simulink model "TST_RailP_DD"  (R2016b)
settings: Solver=FixedStepDiscrete  StartTime=0.0  StopTime=simTime  FixedStep=sampleTime  RelTol=1e-3
values from neighbouring files (symbols this model uses):
  testCase = 1    [initTST_RailP_DD_001.m]    (also in initTST_RailP_DD_002.m = 2; initTST_RailP_DD_003.m = 3)
libraries: UnitTest_Lib x15, simulink x4
settings Model: Creator=liangyunbo  LastModifiedBy=liangyunbo
settings DebuggingCC: SignalRangeChecking=error

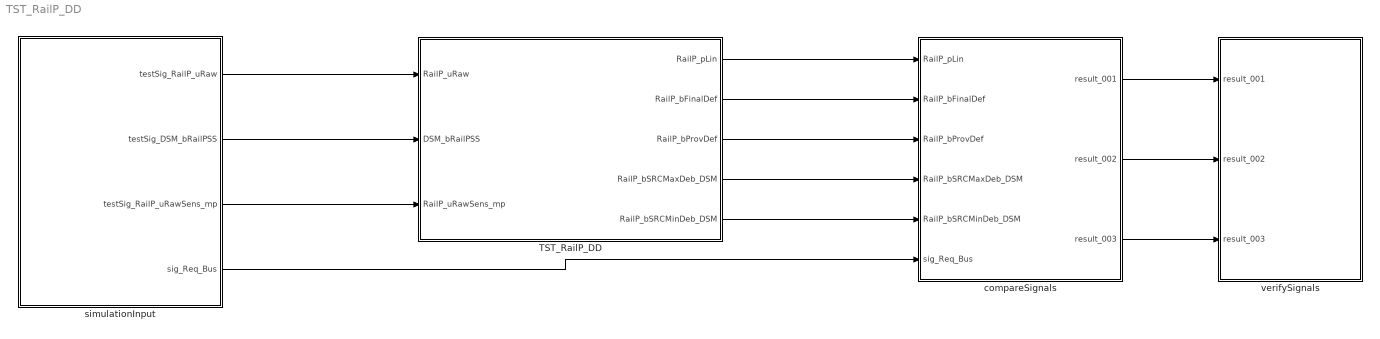
== system TST_RailP_DD ==
  TST_RailP_DD : Subsystem
  compareSignals : Subsystem
  simulationInput : Subsystem
  verifySignals : Subsystem
  wires:
  simulationInput/1(testSig_RailP_uRaw) -> TST_RailP_DD/1(RailP_uRaw)
  simulationInput/2(testSig_DSM_bRailPSS) -> TST_RailP_DD/2(DSM_bRailPSS)
  simulationInput/3(testSig_RailP_uRawSens_mp) -> TST_RailP_DD/3(RailP_uRawSens_mp)
  TST_RailP_DD/1(RailP_pLin) -> compareSignals/1(RailP_pLin)
  TST_RailP_DD/2(RailP_bFinalDef) -> compareSignals/2(RailP_bFinalDef)
  TST_RailP_DD/3(RailP_bProvDef) -> compareSignals/3(RailP_bProvDef)
  TST_RailP_DD/4(RailP_bSRCMaxDeb_DSM) -> compareSignals/4(RailP_bSRCMaxDeb_DSM)
  TST_RailP_DD/5(RailP_bSRCMinDeb_DSM) -> compareSignals/5(RailP_bSRCMinDeb_DSM)
  simulationInput/4(sig_Req_Bus) -> compareSignals/6(sig_Req_Bus)
  compareSignals/1(result_001) -> verifySignals/1(result_001)
  compareSignals/2(result_002) -> verifySignals/2(result_002)
  compareSignals/3(result_003) -> verifySignals/3(result_003)

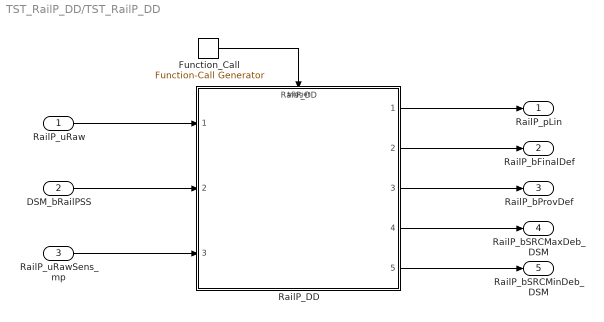
== system TST_RailP_DD/TST_RailP_DD ==
  RailP_uRaw : Inport
  DSM_bRailPSS : Inport  Port=2
  RailP_uRawSens_mp : Inport  Port=3
  Function_Call : simulink/Ports & Subsystems/Function-Call Generator  sample_time=sampleTime  numberOfIterations=1
  RailP_DD : ModelReference  ModelNameDialog=RailP_DD  SimulationMode=Normal  ModelReferenceVersion=1.29  TriggerPortName=function  TriggerPortTriggerType=function-call  TriggerPortStatesWhenEnabling=held
  RailP_pLin : Outport
  RailP_bFinalDef : Outport  Port=2
  RailP_bProvDef : Outport  Port=3
  RailP_bSRCMaxDeb_DSM : Outport  Port=4
  RailP_bSRCMinDeb_DSM : Outport  Port=5
  wires:
  Function_Call/1 -> RailP_DD/Trigger
  RailP_uRaw/1 -> RailP_DD/1
  DSM_bRailPSS/1 -> RailP_DD/2
  RailP_uRawSens_mp/1 -> RailP_DD/3
  RailP_DD/1 -> RailP_pLin/1
  RailP_DD/2 -> RailP_bFinalDef/1
  RailP_DD/3 -> RailP_bProvDef/1
  RailP_DD/4 -> RailP_bSRCMaxDeb_DSM/1
  RailP_DD/5 -> RailP_bSRCMinDeb_DSM/1

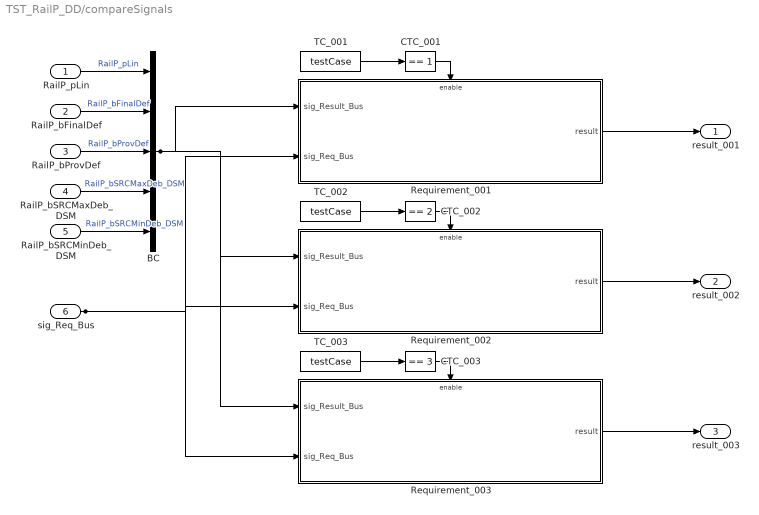
== system TST_RailP_DD/compareSignals ==
  RailP_pLin : Inport
  RailP_bFinalDef : Inport  Port=2
  RailP_bProvDef : Inport  Port=3
  RailP_bSRCMaxDeb_DSM : Inport  Port=4
  RailP_bSRCMinDeb_DSM : Inport  Port=5
  sig_Req_Bus : Inport  Port=6
  BC : BusCreator  Inputs=5
  CTC_001 : simulink/Logic and Bit Operations/Compare To Constant  relop===  const=1  OutDataTypeStr=boolean
  CTC_002 : simulink/Logic and Bit Operations/Compare To Constant  relop===  const=2  OutDataTypeStr=boolean
  CTC_003 : simulink/Logic and Bit Operations/Compare To Constant  relop===  const=3  OutDataTypeStr=boolean
  Requirement_001 : Subsystem
  Requirement_002 : Subsystem
  Requirement_003 : Subsystem
  TC_001 : Constant  Value=testCase
  TC_002 : Constant  Value=testCase
  TC_003 : Constant  Value=testCase
  result_001 : Outport
  result_002 : Outport  Port=2
  result_003 : Outport  Port=3
  wires:
  RailP_pLin/1 -> BC/1  "RailP_pLin"
  RailP_bFinalDef/1 -> BC/2  "RailP_bFinalDef"
  RailP_bProvDef/1 -> BC/3  "RailP_bProvDef"
  RailP_bSRCMaxDeb_DSM/1 -> BC/4  "RailP_bSRCMaxDeb_DSM"
  RailP_bSRCMinDeb_DSM/1 -> BC/5  "RailP_bSRCMinDeb_DSM"
  TC_001/1 -> CTC_001/1
  CTC_001/1 -> Requirement_001/Enable
  sig_Req_Bus/1 -> Requirement_001/2(sig_Req_Bus), Requirement_002/2(sig_Req_Bus), Requirement_003/2(sig_Req_Bus)
  BC/1 -> Requirement_001/1(sig_Result_Bus), Requirement_002/1(sig_Result_Bus), Requirement_003/1(sig_Result_Bus)
  Requirement_001/1(result) -> result_001/1
  TC_002/1 -> CTC_002/1
  CTC_002/1 -> Requirement_002/Enable
  Requirement_002/1(result) -> result_002/1
  TC_003/1 -> CTC_003/1
  CTC_003/1 -> Requirement_003/Enable
  Requirement_003/1(result) -> result_003/1

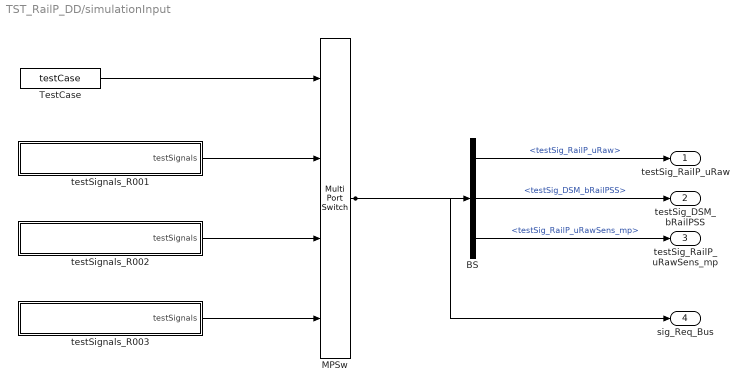
== system TST_RailP_DD/simulationInput ==
  BS : BusSelector  OutputSignals=testSig_RailP_uRaw,testSig_DSM_bRailPSS,testSig_RailP_uRawSens_mp
  MPSw : MultiPortSwitch  SaturateOnIntegerOverflow=on  InputSameDT=on
  TestCase : Constant  Value=testCase
  testSignals_R001 : Subsystem
  testSignals_R002 : Subsystem
  testSignals_R003 : Subsystem
  testSig_RailP_uRaw : Outport
  testSig_DSM_bRailPSS : Outport  Port=2
  testSig_RailP_uRawSens_mp : Outport  Port=3
  sig_Req_Bus : Outport  Port=4
  wires:
  BS/1 -> testSig_RailP_uRaw/1  "<testSig_RailP_uRaw>"
  BS/2 -> testSig_DSM_bRailPSS/1  "<testSig_DSM_bRailPSS>"
  BS/3 -> testSig_RailP_uRawSens_mp/1  "<testSig_RailP_uRawSens_mp>"
  MPSw/1 -> BS/1, sig_Req_Bus/1
  TestCase/1 -> MPSw/1
  testSignals_R001/1(testSignals) -> MPSw/2
  testSignals_R002/1(testSignals) -> MPSw/3
  testSignals_R003/1(testSignals) -> MPSw/4

== system TST_RailP_DD/verifySignals ==
  result_001 : Inport
  result_002 : Inport  Port=2
  result_003 : Inport  Port=3
  Assertion_001 : Assertion  Enabled=off
  Assertion_002 : Assertion  Enabled=off
  Assertion_003 : Assertion  Enabled=off
  wires:
  result_001/1 -> Assertion_001/1
  result_002/1 -> Assertion_002/1
  result_003/1 -> Assertion_003/1

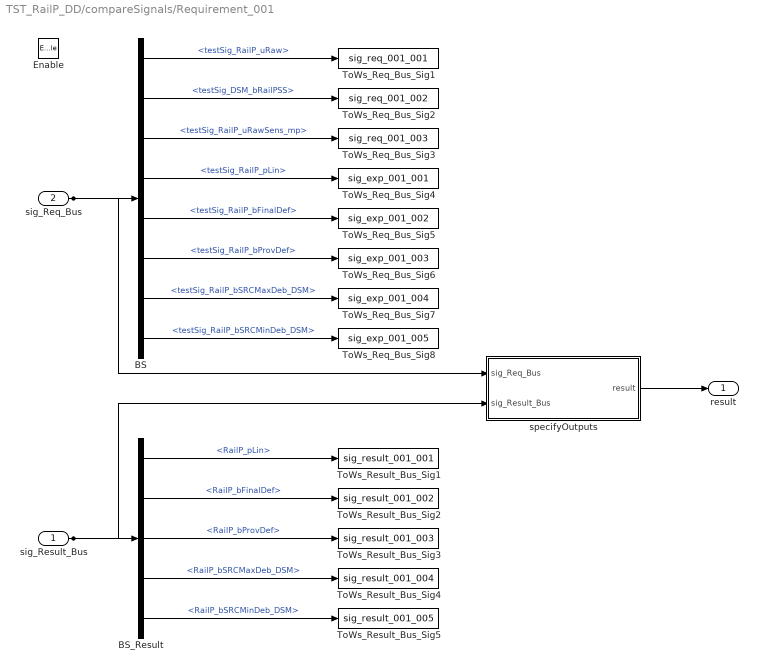
== system TST_RailP_DD/compareSignals/Requirement_001 ==
  sig_Result_Bus : Inport
  sig_Req_Bus : Inport  Port=2
  Enable : EnablePort
  BS : BusSelector  OutputSignals=testSig_RailP_uRaw,testSig_DSM_bRailPSS,testSig_RailP_uRawSens_mp,testSig_RailP_pLin,testSig_RailP_bFinalDef,testSig_RailP_bProvDef,testSig_RailP_bSRCMaxDeb_DSM,testSig_RailP_bSRCMinDeb_DSM
  BS_Result : BusSelector  OutputSignals=RailP_pLin,RailP_bFinalDef,RailP_bProvDef,RailP_bSRCMaxDeb_DSM,RailP_bSRCMinDeb_DSM
  ToWs_Req_Bus_Sig1 : ToWorkspace  VariableName=sig_req_001_001  SaveFormat=Structure With Time
  ToWs_Req_Bus_Sig2 : ToWorkspace  VariableName=sig_req_001_002  SaveFormat=Structure With Time
  ToWs_Req_Bus_Sig3 : ToWorkspace  VariableName=sig_req_001_003  SaveFormat=Structure With Time
  ToWs_Req_Bus_Sig4 : ToWorkspace  VariableName=sig_exp_001_001  SaveFormat=Structure With Time
  ToWs_Req_Bus_Sig5 : ToWorkspace  VariableName=sig_exp_001_002  SaveFormat=Structure With Time
  ToWs_Req_Bus_Sig6 : ToWorkspace  VariableName=sig_exp_001_003  SaveFormat=Structure With Time
  ToWs_Req_Bus_Sig7 : ToWorkspace  VariableName=sig_exp_001_004  SaveFormat=Structure With Time
  ToWs_Req_Bus_Sig8 : ToWorkspace  VariableName=sig_exp_001_005  SaveFormat=Structure With Time
  ToWs_Result_Bus_Sig1 : ToWorkspace  VariableName=sig_result_001_001  SaveFormat=Structure With Time
  ToWs_Result_Bus_Sig2 : ToWorkspace  VariableName=sig_result_001_002  SaveFormat=Structure With Time
  ToWs_Result_Bus_Sig3 : ToWorkspace  VariableName=sig_result_001_003  SaveFormat=Structure With Time
  ToWs_Result_Bus_Sig4 : ToWorkspace  VariableName=sig_result_001_004  SaveFormat=Structure With Time
  ToWs_Result_Bus_Sig5 : ToWorkspace  VariableName=sig_result_001_005  SaveFormat=Structure With Time
  specifyOutputs : Subsystem
  result : Outport
  wires:
  sig_Req_Bus/1 -> BS/1, specifyOutputs/1(sig_Req_Bus)
  BS/1 -> ToWs_Req_Bus_Sig1/1  "<testSig_RailP_uRaw>"
  BS/2 -> ToWs_Req_Bus_Sig2/1  "<testSig_DSM_bRailPSS>"
  BS/3 -> ToWs_Req_Bus_Sig3/1  "<testSig_RailP_uRawSens_mp>"
  BS/4 -> ToWs_Req_Bus_Sig4/1  "<testSig_RailP_pLin>"
  BS/5 -> ToWs_Req_Bus_Sig5/1  "<testSig_RailP_bFinalDef>"
  BS/6 -> ToWs_Req_Bus_Sig6/1  "<testSig_RailP_bProvDef>"
  BS/7 -> ToWs_Req_Bus_Sig7/1  "<testSig_RailP_bSRCMaxDeb_DSM>"
  BS/8 -> ToWs_Req_Bus_Sig8/1  "<testSig_RailP_bSRCMinDeb_DSM>"
  sig_Result_Bus/1 -> BS_Result/1, specifyOutputs/2(sig_Result_Bus)
  BS_Result/1 -> ToWs_Result_Bus_Sig1/1  "<RailP_pLin>"
  BS_Result/2 -> ToWs_Result_Bus_Sig2/1  "<RailP_bFinalDef>"
  BS_Result/3 -> ToWs_Result_Bus_Sig3/1  "<RailP_bProvDef>"
  BS_Result/4 -> ToWs_Result_Bus_Sig4/1  "<RailP_bSRCMaxDeb_DSM>"
  BS_Result/5 -> ToWs_Result_Bus_Sig5/1  "<RailP_bSRCMinDeb_DSM>"
  specifyOutputs/1(result) -> result/1

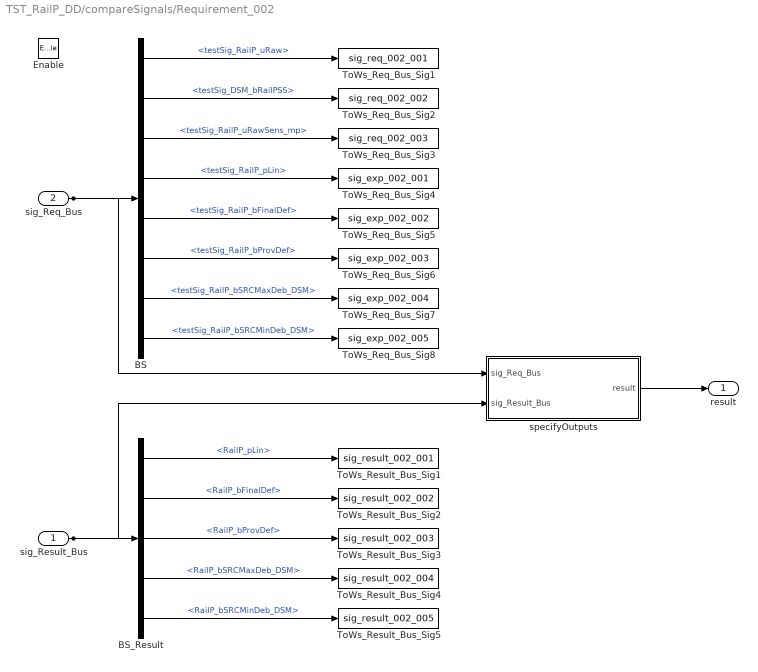
== system TST_RailP_DD/compareSignals/Requirement_002 ==
  sig_Result_Bus : Inport
  sig_Req_Bus : Inport  Port=2
  Enable : EnablePort
  BS : BusSelector  OutputSignals=testSig_RailP_uRaw,testSig_DSM_bRailPSS,testSig_RailP_uRawSens_mp,testSig_RailP_pLin,testSig_RailP_bFinalDef,testSig_RailP_bProvDef,testSig_RailP_bSRCMaxDeb_DSM,testSig_RailP_bSRCMinDeb_DSM
  BS_Result : BusSelector  OutputSignals=RailP_pLin,RailP_bFinalDef,RailP_bProvDef,RailP_bSRCMaxDeb_DSM,RailP_bSRCMinDeb_DSM
  ToWs_Req_Bus_Sig1 : ToWorkspace  VariableName=sig_req_002_001  SaveFormat=Structure With Time
  ToWs_Req_Bus_Sig2 : ToWorkspace  VariableName=sig_req_002_002  SaveFormat=Structure With Time
  ToWs_Req_Bus_Sig3 : ToWorkspace  VariableName=sig_req_002_003  SaveFormat=Structure With Time
  ToWs_Req_Bus_Sig4 : ToWorkspace  VariableName=sig_exp_002_001  SaveFormat=Structure With Time
  ToWs_Req_Bus_Sig5 : ToWorkspace  VariableName=sig_exp_002_002  SaveFormat=Structure With Time
  ToWs_Req_Bus_Sig6 : ToWorkspace  VariableName=sig_exp_002_003  SaveFormat=Structure With Time
  ToWs_Req_Bus_Sig7 : ToWorkspace  VariableName=sig_exp_002_004  SaveFormat=Structure With Time
  ToWs_Req_Bus_Sig8 : ToWorkspace  VariableName=sig_exp_002_005  SaveFormat=Structure With Time
  ToWs_Result_Bus_Sig1 : ToWorkspace  VariableName=sig_result_002_001  SaveFormat=Structure With Time
  ToWs_Result_Bus_Sig2 : ToWorkspace  VariableName=sig_result_002_002  SaveFormat=Structure With Time
  ToWs_Result_Bus_Sig3 : ToWorkspace  VariableName=sig_result_002_003  SaveFormat=Structure With Time
  ToWs_Result_Bus_Sig4 : ToWorkspace  VariableName=sig_result_002_004  SaveFormat=Structure With Time
  ToWs_Result_Bus_Sig5 : ToWorkspace  VariableName=sig_result_002_005  SaveFormat=Structure With Time
  specifyOutputs : Subsystem
  result : Outport
  wires:
  sig_Req_Bus/1 -> BS/1, specifyOutputs/1(sig_Req_Bus)
  BS/1 -> ToWs_Req_Bus_Sig1/1  "<testSig_RailP_uRaw>"
  BS/2 -> ToWs_Req_Bus_Sig2/1  "<testSig_DSM_bRailPSS>"
  BS/3 -> ToWs_Req_Bus_Sig3/1  "<testSig_RailP_uRawSens_mp>"
  BS/4 -> ToWs_Req_Bus_Sig4/1  "<testSig_RailP_pLin>"
  BS/5 -> ToWs_Req_Bus_Sig5/1  "<testSig_RailP_bFinalDef>"
  BS/6 -> ToWs_Req_Bus_Sig6/1  "<testSig_RailP_bProvDef>"
  BS/7 -> ToWs_Req_Bus_Sig7/1  "<testSig_RailP_bSRCMaxDeb_DSM>"
  BS/8 -> ToWs_Req_Bus_Sig8/1  "<testSig_RailP_bSRCMinDeb_DSM>"
  sig_Result_Bus/1 -> BS_Result/1, specifyOutputs/2(sig_Result_Bus)
  BS_Result/1 -> ToWs_Result_Bus_Sig1/1  "<RailP_pLin>"
  BS_Result/2 -> ToWs_Result_Bus_Sig2/1  "<RailP_bFinalDef>"
  BS_Result/3 -> ToWs_Result_Bus_Sig3/1  "<RailP_bProvDef>"
  BS_Result/4 -> ToWs_Result_Bus_Sig4/1  "<RailP_bSRCMaxDeb_DSM>"
  BS_Result/5 -> ToWs_Result_Bus_Sig5/1  "<RailP_bSRCMinDeb_DSM>"
  specifyOutputs/1(result) -> result/1

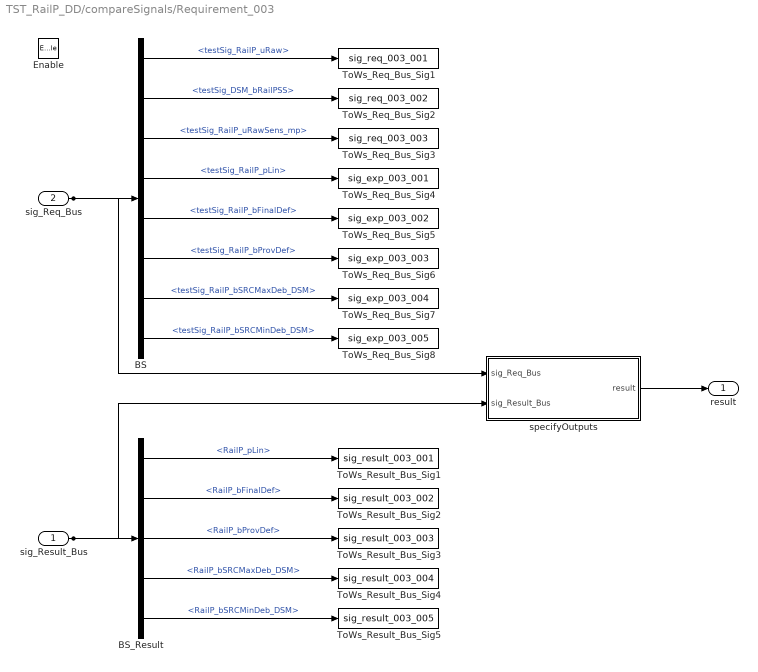
== system TST_RailP_DD/compareSignals/Requirement_003 ==
  sig_Result_Bus : Inport
  sig_Req_Bus : Inport  Port=2
  Enable : EnablePort
  BS : BusSelector  OutputSignals=testSig_RailP_uRaw,testSig_DSM_bRailPSS,testSig_RailP_uRawSens_mp,testSig_RailP_pLin,testSig_RailP_bFinalDef,testSig_RailP_bProvDef,testSig_RailP_bSRCMaxDeb_DSM,testSig_RailP_bSRCMinDeb_DSM
  BS_Result : BusSelector  OutputSignals=RailP_pLin,RailP_bFinalDef,RailP_bProvDef,RailP_bSRCMaxDeb_DSM,RailP_bSRCMinDeb_DSM
  ToWs_Req_Bus_Sig1 : ToWorkspace  VariableName=sig_req_003_001  SaveFormat=Structure With Time
  ToWs_Req_Bus_Sig2 : ToWorkspace  VariableName=sig_req_003_002  SaveFormat=Structure With Time
  ToWs_Req_Bus_Sig3 : ToWorkspace  VariableName=sig_req_003_003  SaveFormat=Structure With Time
  ToWs_Req_Bus_Sig4 : ToWorkspace  VariableName=sig_exp_003_001  SaveFormat=Structure With Time
  ToWs_Req_Bus_Sig5 : ToWorkspace  VariableName=sig_exp_003_002  SaveFormat=Structure With Time
  ToWs_Req_Bus_Sig6 : ToWorkspace  VariableName=sig_exp_003_003  SaveFormat=Structure With Time
  ToWs_Req_Bus_Sig7 : ToWorkspace  VariableName=sig_exp_003_004  SaveFormat=Structure With Time
  ToWs_Req_Bus_Sig8 : ToWorkspace  VariableName=sig_exp_003_005  SaveFormat=Structure With Time
  ToWs_Result_Bus_Sig1 : ToWorkspace  VariableName=sig_result_003_001  SaveFormat=Structure With Time
  ToWs_Result_Bus_Sig2 : ToWorkspace  VariableName=sig_result_003_002  SaveFormat=Structure With Time
  ToWs_Result_Bus_Sig3 : ToWorkspace  VariableName=sig_result_003_003  SaveFormat=Structure With Time
  ToWs_Result_Bus_Sig4 : ToWorkspace  VariableName=sig_result_003_004  SaveFormat=Structure With Time
  ToWs_Result_Bus_Sig5 : ToWorkspace  VariableName=sig_result_003_005  SaveFormat=Structure With Time
  specifyOutputs : Subsystem
  result : Outport
  wires:
  sig_Req_Bus/1 -> BS/1, specifyOutputs/1(sig_Req_Bus)
  BS/1 -> ToWs_Req_Bus_Sig1/1  "<testSig_RailP_uRaw>"
  BS/2 -> ToWs_Req_Bus_Sig2/1  "<testSig_DSM_bRailPSS>"
  BS/3 -> ToWs_Req_Bus_Sig3/1  "<testSig_RailP_uRawSens_mp>"
  BS/4 -> ToWs_Req_Bus_Sig4/1  "<testSig_RailP_pLin>"
  BS/5 -> ToWs_Req_Bus_Sig5/1  "<testSig_RailP_bFinalDef>"
  BS/6 -> ToWs_Req_Bus_Sig6/1  "<testSig_RailP_bProvDef>"
  BS/7 -> ToWs_Req_Bus_Sig7/1  "<testSig_RailP_bSRCMaxDeb_DSM>"
  BS/8 -> ToWs_Req_Bus_Sig8/1  "<testSig_RailP_bSRCMinDeb_DSM>"
  sig_Result_Bus/1 -> BS_Result/1, specifyOutputs/2(sig_Result_Bus)
  BS_Result/1 -> ToWs_Result_Bus_Sig1/1  "<RailP_pLin>"
  BS_Result/2 -> ToWs_Result_Bus_Sig2/1  "<RailP_bFinalDef>"
  BS_Result/3 -> ToWs_Result_Bus_Sig3/1  "<RailP_bProvDef>"
  BS_Result/4 -> ToWs_Result_Bus_Sig4/1  "<RailP_bSRCMaxDeb_DSM>"
  BS_Result/5 -> ToWs_Result_Bus_Sig5/1  "<RailP_bSRCMinDeb_DSM>"
  specifyOutputs/1(result) -> result/1

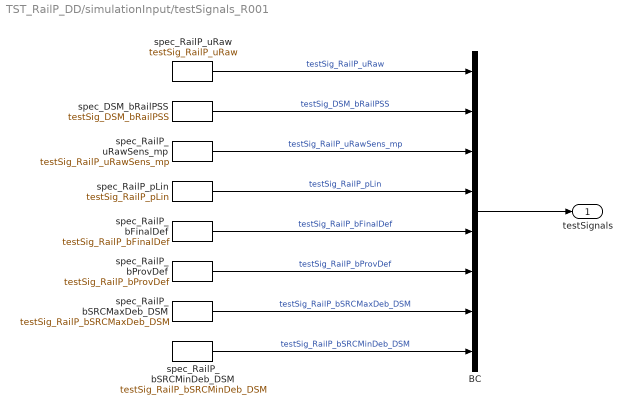
== system TST_RailP_DD/simulationInput/testSignals_R001 ==
  BC : BusCreator  Inputs=8
  spec_DSM_bRailPSS : FromWorkspace  VariableName=testSig_DSM_bRailPSS  Interpolate=off  OutputAfterFinalValue=Holding final value
  spec_RailP_bFinalDef : FromWorkspace  VariableName=testSig_RailP_bFinalDef  Interpolate=off  OutputAfterFinalValue=Holding final value
  spec_RailP_bProvDef : FromWorkspace  VariableName=testSig_RailP_bProvDef  Interpolate=off  OutputAfterFinalValue=Holding final value
  spec_RailP_bSRCMaxDeb_DSM : FromWorkspace  VariableName=testSig_RailP_bSRCMaxDeb_DSM  Interpolate=off  OutputAfterFinalValue=Holding final value
  spec_RailP_bSRCMinDeb_DSM : FromWorkspace  VariableName=testSig_RailP_bSRCMinDeb_DSM  Interpolate=off  OutputAfterFinalValue=Holding final value
  spec_RailP_pLin : FromWorkspace  VariableName=testSig_RailP_pLin  Interpolate=off  OutputAfterFinalValue=Holding final value
  spec_RailP_uRaw : FromWorkspace  VariableName=testSig_RailP_uRaw  Interpolate=off  OutputAfterFinalValue=Holding final value
  spec_RailP_uRawSens_mp : FromWorkspace  VariableName=testSig_RailP_uRawSens_mp  Interpolate=off  OutputAfterFinalValue=Holding final value
  testSignals : Outport
  wires:
  BC/1 -> testSignals/1
  spec_RailP_uRaw/1 -> BC/1  "testSig_RailP_uRaw"
  spec_DSM_bRailPSS/1 -> BC/2  "testSig_DSM_bRailPSS"
  spec_RailP_uRawSens_mp/1 -> BC/3  "testSig_RailP_uRawSens_mp"
  spec_RailP_pLin/1 -> BC/4  "testSig_RailP_pLin"
  spec_RailP_bFinalDef/1 -> BC/5  "testSig_RailP_bFinalDef"
  spec_RailP_bProvDef/1 -> BC/6  "testSig_RailP_bProvDef"
  spec_RailP_bSRCMaxDeb_DSM/1 -> BC/7  "testSig_RailP_bSRCMaxDeb_DSM"
  spec_RailP_bSRCMinDeb_DSM/1 -> BC/8  "testSig_RailP_bSRCMinDeb_DSM"

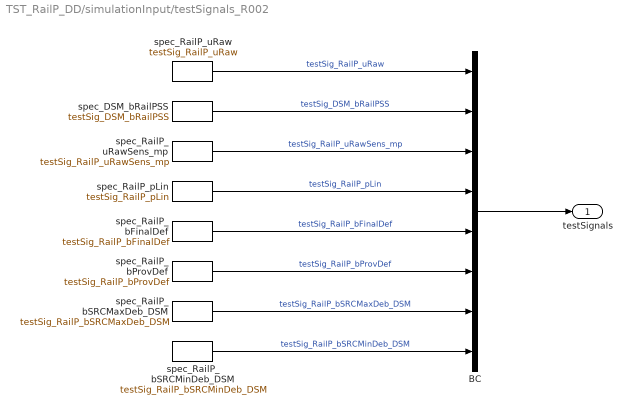
== system TST_RailP_DD/simulationInput/testSignals_R002 ==
  BC : BusCreator  Inputs=8
  spec_DSM_bRailPSS : FromWorkspace  VariableName=testSig_DSM_bRailPSS  Interpolate=off  OutputAfterFinalValue=Holding final value
  spec_RailP_bFinalDef : FromWorkspace  VariableName=testSig_RailP_bFinalDef  Interpolate=off  OutputAfterFinalValue=Holding final value
  spec_RailP_bProvDef : FromWorkspace  VariableName=testSig_RailP_bProvDef  Interpolate=off  OutputAfterFinalValue=Holding final value
  spec_RailP_bSRCMaxDeb_DSM : FromWorkspace  VariableName=testSig_RailP_bSRCMaxDeb_DSM  Interpolate=off  OutputAfterFinalValue=Holding final value
  spec_RailP_bSRCMinDeb_DSM : FromWorkspace  VariableName=testSig_RailP_bSRCMinDeb_DSM  Interpolate=off  OutputAfterFinalValue=Holding final value
  spec_RailP_pLin : FromWorkspace  VariableName=testSig_RailP_pLin  Interpolate=off  OutputAfterFinalValue=Holding final value
  spec_RailP_uRaw : FromWorkspace  VariableName=testSig_RailP_uRaw  Interpolate=off  OutputAfterFinalValue=Holding final value
  spec_RailP_uRawSens_mp : FromWorkspace  VariableName=testSig_RailP_uRawSens_mp  Interpolate=off  OutputAfterFinalValue=Holding final value
  testSignals : Outport
  wires:
  BC/1 -> testSignals/1
  spec_RailP_uRaw/1 -> BC/1  "testSig_RailP_uRaw"
  spec_DSM_bRailPSS/1 -> BC/2  "testSig_DSM_bRailPSS"
  spec_RailP_uRawSens_mp/1 -> BC/3  "testSig_RailP_uRawSens_mp"
  spec_RailP_pLin/1 -> BC/4  "testSig_RailP_pLin"
  spec_RailP_bFinalDef/1 -> BC/5  "testSig_RailP_bFinalDef"
  spec_RailP_bProvDef/1 -> BC/6  "testSig_RailP_bProvDef"
  spec_RailP_bSRCMaxDeb_DSM/1 -> BC/7  "testSig_RailP_bSRCMaxDeb_DSM"
  spec_RailP_bSRCMinDeb_DSM/1 -> BC/8  "testSig_RailP_bSRCMinDeb_DSM"

== system TST_RailP_DD/simulationInput/testSignals_R003 ==
  BC : BusCreator  Inputs=8
  spec_DSM_bRailPSS : FromWorkspace  VariableName=testSig_DSM_bRailPSS  Interpolate=off  OutputAfterFinalValue=Holding final value
  spec_RailP_bFinalDef : FromWorkspace  VariableName=testSig_RailP_bFinalDef  Interpolate=off  OutputAfterFinalValue=Holding final value
  spec_RailP_bProvDef : FromWorkspace  VariableName=testSig_RailP_bProvDef  Interpolate=off  OutputAfterFinalValue=Holding final value
  spec_RailP_bSRCMaxDeb_DSM : FromWorkspace  VariableName=testSig_RailP_bSRCMaxDeb_DSM  Interpolate=off  OutputAfterFinalValue=Holding final value
  spec_RailP_bSRCMinDeb_DSM : FromWorkspace  VariableName=testSig_RailP_bSRCMinDeb_DSM  Interpolate=off  OutputAfterFinalValue=Holding final value
  spec_RailP_pLin : FromWorkspace  VariableName=testSig_RailP_pLin  Interpolate=off  OutputAfterFinalValue=Holding final value
  spec_RailP_uRaw : FromWorkspace  VariableName=testSig_RailP_uRaw  Interpolate=off  OutputAfterFinalValue=Holding final value
  spec_RailP_uRawSens_mp : FromWorkspace  VariableName=testSig_RailP_uRawSens_mp  Interpolate=off  OutputAfterFinalValue=Holding final value
  testSignals : Outport
  wires:
  BC/1 -> testSignals/1
  spec_RailP_uRaw/1 -> BC/1  "testSig_RailP_uRaw"
  spec_DSM_bRailPSS/1 -> BC/2  "testSig_DSM_bRailPSS"
  spec_RailP_uRawSens_mp/1 -> BC/3  "testSig_RailP_uRawSens_mp"
  spec_RailP_pLin/1 -> BC/4  "testSig_RailP_pLin"
  spec_RailP_bFinalDef/1 -> BC/5  "testSig_RailP_bFinalDef"
  spec_RailP_bProvDef/1 -> BC/6  "testSig_RailP_bProvDef"
  spec_RailP_bSRCMaxDeb_DSM/1 -> BC/7  "testSig_RailP_bSRCMaxDeb_DSM"
  spec_RailP_bSRCMinDeb_DSM/1 -> BC/8  "testSig_RailP_bSRCMinDeb_DSM"

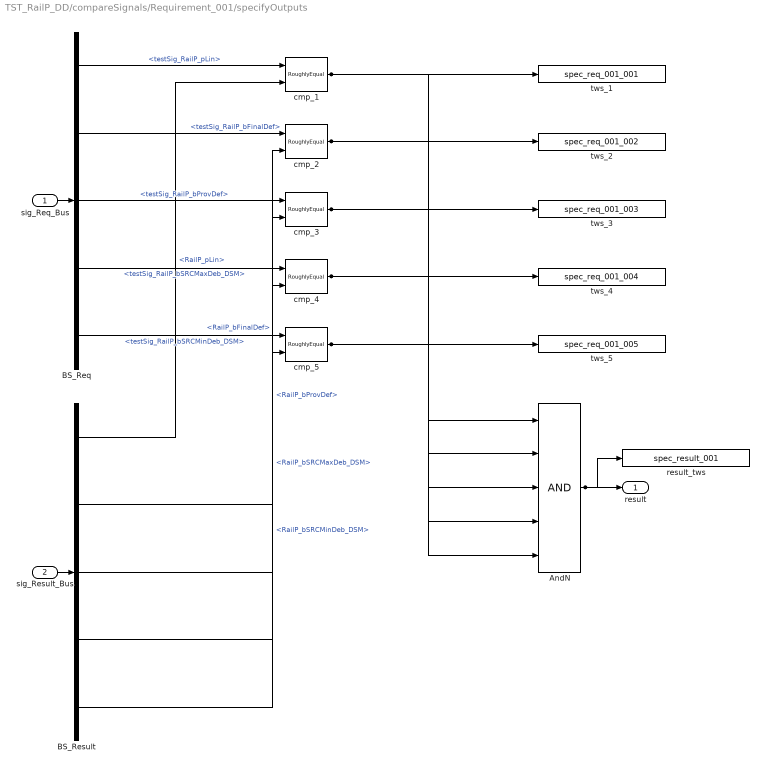
== system TST_RailP_DD/compareSignals/Requirement_001/specifyOutputs ==
  sig_Req_Bus : Inport
  sig_Result_Bus : Inport  Port=2
  AndN : Logic  Inputs=5
  BS_Req : BusSelector  OutputSignals=testSig_RailP_pLin,testSig_RailP_bFinalDef,testSig_RailP_bProvDef,testSig_RailP_bSRCMaxDeb_DSM,testSig_RailP_bSRCMinDeb_DSM
  BS_Result : BusSelector  OutputSignals=RailP_pLin,RailP_bFinalDef,RailP_bProvDef,RailP_bSRCMaxDeb_DSM,RailP_bSRCMinDeb_DSM
  cmp_{1..5} (5 alike) : UnitTest_Lib/RoughlyEqual  slope=0.1
  result_tws : ToWorkspace  VariableName=spec_result_001
  tws_1 : ToWorkspace  VariableName=spec_req_001_001
  tws_2 : ToWorkspace  VariableName=spec_req_001_002
  tws_3 : ToWorkspace  VariableName=spec_req_001_003
  tws_4 : ToWorkspace  VariableName=spec_req_001_004
  tws_5 : ToWorkspace  VariableName=spec_req_001_005
  result : Outport
  wires:
  sig_Req_Bus/1 -> BS_Req/1
  sig_Result_Bus/1 -> BS_Result/1
  AndN/1 -> result/1, result_tws/1
  BS_Req/1 -> cmp_1/1  "<testSig_RailP_pLin>"
  BS_Result/1 -> cmp_1/2  "<RailP_pLin>"
  cmp_1/1 -> tws_1/1, AndN/1
  BS_Req/2 -> cmp_2/1  "<testSig_RailP_bFinalDef>"
  BS_Result/2 -> cmp_2/2  "<RailP_bFinalDef>"
  cmp_2/1 -> tws_2/1, AndN/2
  BS_Req/3 -> cmp_3/1  "<testSig_RailP_bProvDef>"
  BS_Result/3 -> cmp_3/2  "<RailP_bProvDef>"
  cmp_3/1 -> tws_3/1, AndN/3
  BS_Req/4 -> cmp_4/1  "<testSig_RailP_bSRCMaxDeb_DSM>"
  BS_Result/4 -> cmp_4/2  "<RailP_bSRCMaxDeb_DSM>"
  cmp_4/1 -> tws_4/1, AndN/4
  BS_Req/5 -> cmp_5/1  "<testSig_RailP_bSRCMinDeb_DSM>"
  BS_Result/5 -> cmp_5/2  "<RailP_bSRCMinDeb_DSM>"
  cmp_5/1 -> tws_5/1, AndN/5

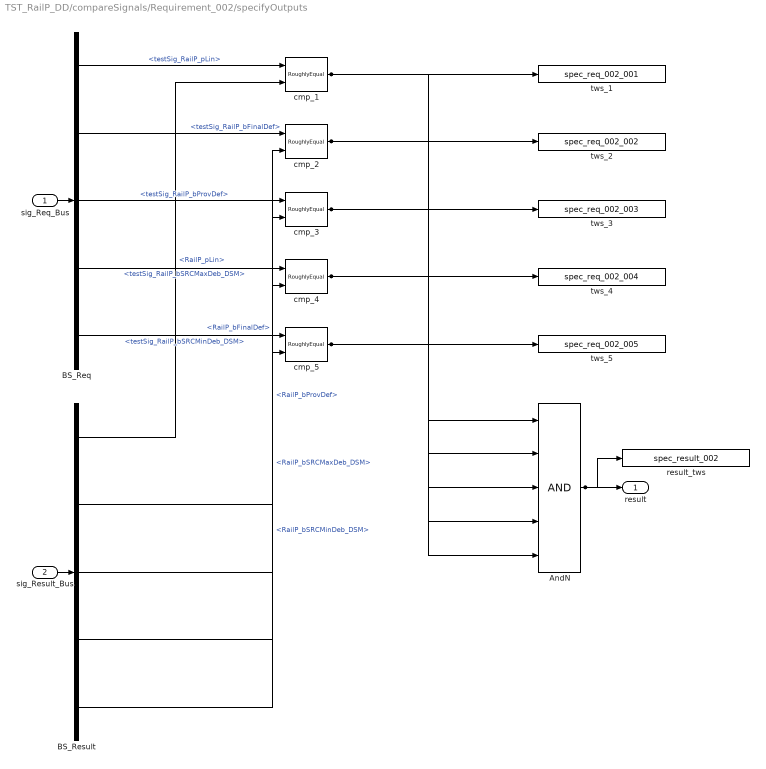
== system TST_RailP_DD/compareSignals/Requirement_002/specifyOutputs ==
  sig_Req_Bus : Inport
  sig_Result_Bus : Inport  Port=2
  AndN : Logic  Inputs=5
  BS_Req : BusSelector  OutputSignals=testSig_RailP_pLin,testSig_RailP_bFinalDef,testSig_RailP_bProvDef,testSig_RailP_bSRCMaxDeb_DSM,testSig_RailP_bSRCMinDeb_DSM
  BS_Result : BusSelector  OutputSignals=RailP_pLin,RailP_bFinalDef,RailP_bProvDef,RailP_bSRCMaxDeb_DSM,RailP_bSRCMinDeb_DSM
  cmp_{1..5} (5 alike) : UnitTest_Lib/RoughlyEqual  slope=0.1
  result_tws : ToWorkspace  VariableName=spec_result_002
  tws_1 : ToWorkspace  VariableName=spec_req_002_001
  tws_2 : ToWorkspace  VariableName=spec_req_002_002
  tws_3 : ToWorkspace  VariableName=spec_req_002_003
  tws_4 : ToWorkspace  VariableName=spec_req_002_004
  tws_5 : ToWorkspace  VariableName=spec_req_002_005
  result : Outport
  wires:
  sig_Req_Bus/1 -> BS_Req/1
  sig_Result_Bus/1 -> BS_Result/1
  AndN/1 -> result/1, result_tws/1
  BS_Req/1 -> cmp_1/1  "<testSig_RailP_pLin>"
  BS_Result/1 -> cmp_1/2  "<RailP_pLin>"
  cmp_1/1 -> tws_1/1, AndN/1
  BS_Req/2 -> cmp_2/1  "<testSig_RailP_bFinalDef>"
  BS_Result/2 -> cmp_2/2  "<RailP_bFinalDef>"
  cmp_2/1 -> tws_2/1, AndN/2
  BS_Req/3 -> cmp_3/1  "<testSig_RailP_bProvDef>"
  BS_Result/3 -> cmp_3/2  "<RailP_bProvDef>"
  cmp_3/1 -> tws_3/1, AndN/3
  BS_Req/4 -> cmp_4/1  "<testSig_RailP_bSRCMaxDeb_DSM>"
  BS_Result/4 -> cmp_4/2  "<RailP_bSRCMaxDeb_DSM>"
  cmp_4/1 -> tws_4/1, AndN/4
  BS_Req/5 -> cmp_5/1  "<testSig_RailP_bSRCMinDeb_DSM>"
  BS_Result/5 -> cmp_5/2  "<RailP_bSRCMinDeb_DSM>"
  cmp_5/1 -> tws_5/1, AndN/5

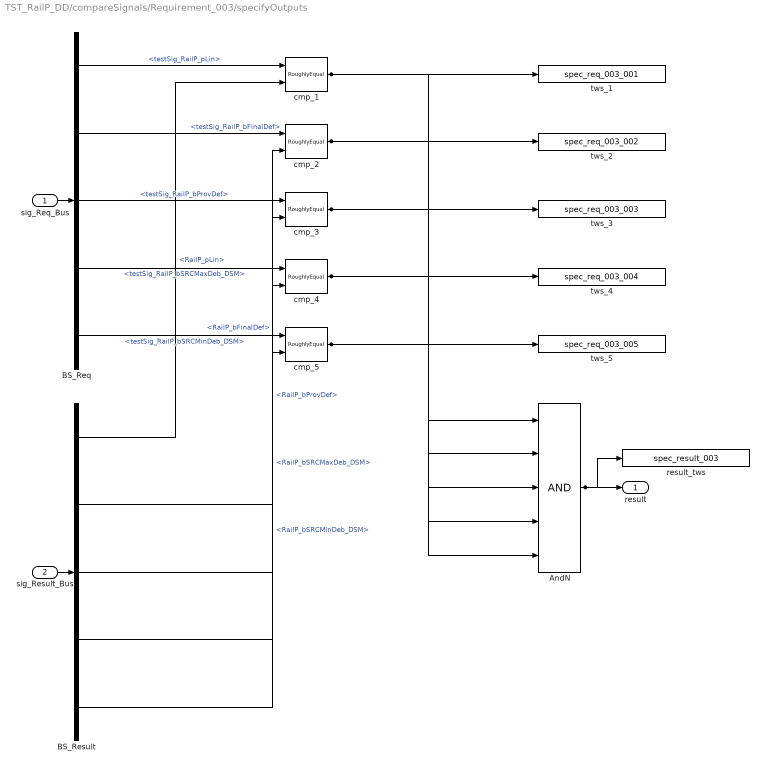
== system TST_RailP_DD/compareSignals/Requirement_003/specifyOutputs ==
  sig_Req_Bus : Inport
  sig_Result_Bus : Inport  Port=2
  AndN : Logic  Inputs=5
  BS_Req : BusSelector  OutputSignals=testSig_RailP_pLin,testSig_RailP_bFinalDef,testSig_RailP_bProvDef,testSig_RailP_bSRCMaxDeb_DSM,testSig_RailP_bSRCMinDeb_DSM
  BS_Result : BusSelector  OutputSignals=RailP_pLin,RailP_bFinalDef,RailP_bProvDef,RailP_bSRCMaxDeb_DSM,RailP_bSRCMinDeb_DSM
  cmp_{1..5} (5 alike) : UnitTest_Lib/RoughlyEqual  slope=0.1
  result_tws : ToWorkspace  VariableName=spec_result_003
  tws_1 : ToWorkspace  VariableName=spec_req_003_001
  tws_2 : ToWorkspace  VariableName=spec_req_003_002
  tws_3 : ToWorkspace  VariableName=spec_req_003_003
  tws_4 : ToWorkspace  VariableName=spec_req_003_004
  tws_5 : ToWorkspace  VariableName=spec_req_003_005
  result : Outport
  wires:
  sig_Req_Bus/1 -> BS_Req/1
  sig_Result_Bus/1 -> BS_Result/1
  AndN/1 -> result/1, result_tws/1
  BS_Req/1 -> cmp_1/1  "<testSig_RailP_pLin>"
  BS_Result/1 -> cmp_1/2  "<RailP_pLin>"
  cmp_1/1 -> tws_1/1, AndN/1
  BS_Req/2 -> cmp_2/1  "<testSig_RailP_bFinalDef>"
  BS_Result/2 -> cmp_2/2  "<RailP_bFinalDef>"
  cmp_2/1 -> tws_2/1, AndN/2
  BS_Req/3 -> cmp_3/1  "<testSig_RailP_bProvDef>"
  BS_Result/3 -> cmp_3/2  "<RailP_bProvDef>"
  cmp_3/1 -> tws_3/1, AndN/3
  BS_Req/4 -> cmp_4/1  "<testSig_RailP_bSRCMaxDeb_DSM>"
  BS_Result/4 -> cmp_4/2  "<RailP_bSRCMaxDeb_DSM>"
  cmp_4/1 -> tws_4/1, AndN/4
  BS_Req/5 -> cmp_5/1  "<testSig_RailP_bSRCMinDeb_DSM>"
  BS_Result/5 -> cmp_5/2  "<RailP_bSRCMinDeb_DSM>"
  cmp_5/1 -> tws_5/1, AndN/5
